simulink model "current"  (R2016b)
settings: Solver=VariableStepAuto  StartTime=0.0  StopTime=0.15  FixedStep=1e-5  MaxStep=Ts  RelTol=1e-4
model workspace (MAT data in the model file):
  TL = 0
  Ti = 0.001
  fpwm = 5000
  ts = 2e-06
undefined symbols (not defined in the file): Kii, Kpi, pmsm, Ts
libraries: nesl_utility x11, fl_lib x9, pe_lib x4, simulink x3, elec_lib x1, pePwmGeneratorTwoLevel x1
settings Model: Creator=25097  LastModifiedBy=25097
settings DebuggingCC: AlgebraicLoopMsg=error  ArtificialAlgebraicLoopMsg=error

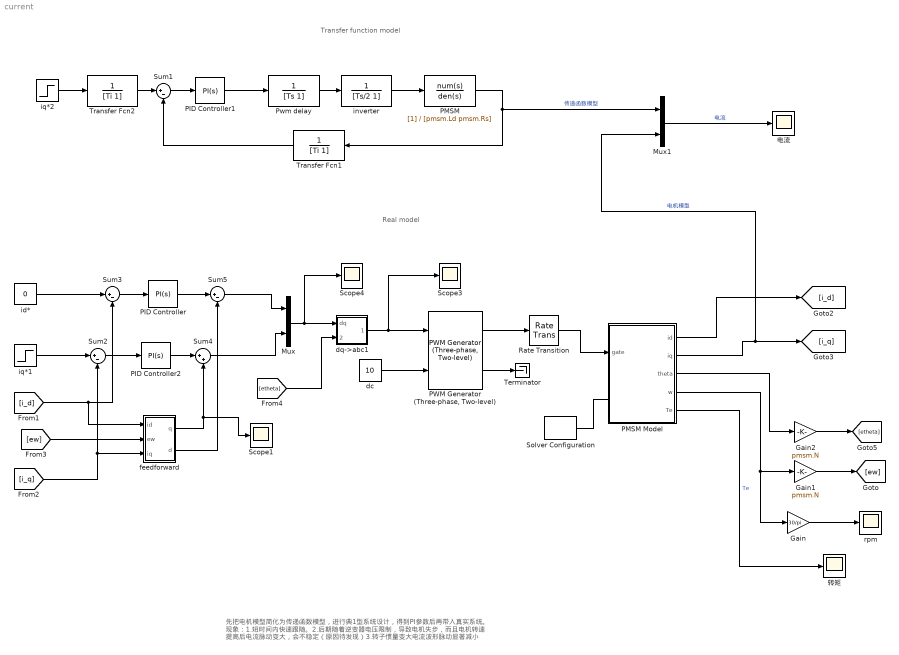
== system current ==
  note: 先把电机模型简化为传递函数模型，进行典1型系统设计，得到PI参数后再带入真实系统。
      | 现象：1.短时间内快速跟随。2.后期随着逆变器电压限制，导致电机失步，而且电机转速
      | 提高后电流脉动变大，会不稳定（原因待发现）3.转子惯量变大电流波形脉动显著减小
  note: Transfer function model
  note: Real model
  Gain : Gain  Gain=30/pi
  Gain1 : Gain  Gain=pmsm.N
  Gain2 : Gain  Gain=pmsm.N
  Mux : Mux  Inputs=2
  Mux1 : Mux  Inputs=2
  PID Controller : simulink/Continuous/PID Controller  Controller=PI  TimeDomain=Continuous-time  SampleTime=-1  IntegratorMethod=Forward Euler  FilterMethod=Forward Euler  Form=Parallel  UseFilter=on  ControllerParametersSource=internal  P=Kpi  I=Kii  D=0  N=100  InitialConditionSource=internal  InitialConditionForIntegrator=0  InitialConditionForFilter=0  ExternalReset=none  LimitOutput=off  UpperSaturationLimit=inf  LowerSaturationLimit=-inf  LinearizeAsGain=on  AntiWindupMode=none  Kb=1  TrackingMode=off  Kt=1  PParamMin=[]  PParamMax=[]  IParamMin=[]  IParamMax=[]  DParamMin=[]  DParamMax=[]  NParamMin=[]  NParamMax=[]  KbParamMin=[]  KbParamMax=[]  KtParamMin=[]  KtParamMax=[]  POutMin=[]  POutMax=[]  IOutMin=[]  IOutMax=[]  DOutMin=[]  DOutMax=[]  NOutMin=[]  NOutMax=[]  KbOutMin=[]  KbOutMax=[]  KtOutMin=[]  KtOutMax=[]  IntegratorOutMin=[]  IntegratorOutMax=[]  FilterOutMin=[]  FilterOutMax=[]  SumOutMin=[]  SumOutMax=[]  SumI1OutMin=[]  SumI1OutMax=[]  SumI2OutMin=[]  SumI2OutMax=[]  SumI3OutMin=[]  SumI3OutMax=[]  SumDOutMin=[]  SumDOutMax=[]  SaturationOutMin=[]  SaturationOutMax=[]  IntegratorContinuousStateAttributes=''  IntegratorStateMustResolveToSignalObject=off  IntegratorRTWStateStorageClass=Auto  FilterContinuousStateAttributes=''  FilterStateMustResolveToSignalObject=off  FilterRTWStateStorageClass=Auto  DifferentiatorICPrevScaledInput=0  DifferentiatorOutMin=[]  DifferentiatorOutMax=[]
  PID Controller1 : simulink/Continuous/PID Controller  Controller=PI  TimeDomain=Continuous-time  SampleTime=-1  IntegratorMethod=Forward Euler  FilterMethod=Forward Euler  Form=Parallel  UseFilter=on  ControllerParametersSource=internal  P=Kpi  I=Kii  D=0  N=100  InitialConditionSource=internal  InitialConditionForIntegrator=0  InitialConditionForFilter=0  ExternalReset=none  LimitOutput=off  UpperSaturationLimit=5  LowerSaturationLimit=-5  LinearizeAsGain=on  AntiWindupMode=none  Kb=1  TrackingMode=off  Kt=1  PParamMin=[]  PParamMax=[]  IParamMin=[]  IParamMax=[]  DParamMin=[]  DParamMax=[]  NParamMin=[]  NParamMax=[]  KbParamMin=[]  KbParamMax=[]  KtParamMin=[]  KtParamMax=[]  POutMin=[]  POutMax=[]  IOutMin=[]  IOutMax=[]  DOutMin=[]  DOutMax=[]  NOutMin=[]  NOutMax=[]  KbOutMin=[]  KbOutMax=[]  KtOutMin=[]  KtOutMax=[]  IntegratorOutMin=[]  IntegratorOutMax=[]  FilterOutMin=[]  FilterOutMax=[]  SumOutMin=[]  SumOutMax=[]  SumI1OutMin=[]  SumI1OutMax=[]  SumI2OutMin=[]  SumI2OutMax=[]  SumI3OutMin=[]  SumI3OutMax=[]  SumDOutMin=[]  SumDOutMax=[]  SaturationOutMin=[]  SaturationOutMax=[]  IntegratorContinuousStateAttributes=''  IntegratorStateMustResolveToSignalObject=off  IntegratorRTWStateStorageClass=Auto  FilterContinuousStateAttributes=''  FilterStateMustResolveToSignalObject=off  FilterRTWStateStorageClass=Auto  DifferentiatorICPrevScaledInput=0  DifferentiatorOutMin=[]  DifferentiatorOutMax=[]
  PID Controller2 : simulink/Continuous/PID Controller  Controller=PI  TimeDomain=Continuous-time  SampleTime=-1  IntegratorMethod=Forward Euler  FilterMethod=Forward Euler  Form=Parallel  UseFilter=on  ControllerParametersSource=internal  P=Kpi  I=Kii  D=0  N=100  InitialConditionSource=internal  InitialConditionForIntegrator=0  InitialConditionForFilter=0  ExternalReset=none  LimitOutput=off  UpperSaturationLimit=inf  LowerSaturationLimit=-inf  LinearizeAsGain=on  AntiWindupMode=none  Kb=1  TrackingMode=off  Kt=1  PParamMin=[]  PParamMax=[]  IParamMin=[]  IParamMax=[]  DParamMin=[]  DParamMax=[]  NParamMin=[]  NParamMax=[]  KbParamMin=[]  KbParamMax=[]  KtParamMin=[]  KtParamMax=[]  POutMin=[]  POutMax=[]  IOutMin=[]  IOutMax=[]  DOutMin=[]  DOutMax=[]  NOutMin=[]  NOutMax=[]  KbOutMin=[]  KbOutMax=[]  KtOutMin=[]  KtOutMax=[]  IntegratorOutMin=[]  IntegratorOutMax=[]  FilterOutMin=[]  FilterOutMax=[]  SumOutMin=[]  SumOutMax=[]  SumI1OutMin=[]  SumI1OutMax=[]  SumI2OutMin=[]  SumI2OutMax=[]  SumI3OutMin=[]  SumI3OutMax=[]  SumDOutMin=[]  SumDOutMax=[]  SaturationOutMin=[]  SaturationOutMax=[]  IntegratorContinuousStateAttributes=''  IntegratorStateMustResolveToSignalObject=off  IntegratorRTWStateStorageClass=Auto  FilterContinuousStateAttributes=''  FilterStateMustResolveToSignalObject=off  FilterRTWStateStorageClass=Auto  DifferentiatorICPrevScaledInput=0  DifferentiatorOutMin=[]  DifferentiatorOutMax=[]
  "PMSM " : TransferFcn  Denominator=[pmsm.Ld pmsm.Rs]
  PMSM Model : Subsystem
      settings: MinAlgLoopOccurrences=on
  "PWM Generator (Three-phase, Two-level)" : pePwmGeneratorTwoLevel/PWM Generator (Three-phase, Two-level)  OverrideUsingVariant=NaturalMode  PWMMode=Continuous PWM (CPWM)  CPWMMode=SPWM: sinusoidal PWM  DPWMMode=60 DPWM: 60 degree discontinuous PWM  fsw=fpwm  Ts=ts
      settings: SamplingMode=Natural
  "Pwm delay " : TransferFcn  Denominator=[Ts 1]
  Rate Transition : RateTransition
  Scope1 : Scope
  Scope3 : Scope
  Scope4 : Scope
  Solver Configuration : nesl_utility/Solver Configuration  PhysicalDomain=network_engine_domain  SubClassName=solver  LeftPortType=input  RightPortType=generic  Accelerate=off  Tones=[]  Harmonics=[]  SimulateNoise=off  Profile=off  UseLocalSampling=off  EnableSwitchedLinearOptims=on  FrequencyDomain=off  UseCCode=off  RelTol=0.001  AbsTol=1e-06  MinStep=1e-09  ToWorkspace=off  RevertToSquareIcSolve=off  NumHomotopyIterations=100  PhasorMode=off  PhasorModeNumHarmonics=1  OverrideAbsTol=off  DoDC=off  ResidualTolerance=1e-07  UseLocalSolver=off  LocalSolverChoice=NE_BACKWARD_EULER_ADVANCER  LocalSolverSampleTime=1e-6  DoFixedCost=off  MaxNonlinIter=3  MaxModeIter=2  LinearAlgebra=Sparse  DelaysMemoryBudget=1024  AutomaticFiltering=on  FilteringTimeConstant=0.001
  Sum{1..3,5} (4 alike) : Sum  Inputs=|+-
  Sum4 : Sum  Inputs=|++
  Terminator : Terminator
  Transfer Fcn1 : TransferFcn  Denominator=[Ti 1]
  Transfer Fcn2 : TransferFcn  Denominator=[Ti 1]
  dc : Constant  Value=10
  dq->abc1 : Subsystem
  "feedforward " : Subsystem
  id* : Constant  Value=0
  inverter : TransferFcn  Denominator=[Ts/2 1]
  iq*1 : Step  Time=0.05  After=3  SampleTime=0
  iq*2 : Step  Time=0.05  After=3  SampleTime=0
  rpm : Scope
  电流 : Scope
  转矩 : Scope
  wires:
  iq*2/1 -> Transfer Fcn2/1
  Transfer Fcn2/1 -> Sum1/1
  Sum1/1 -> PID Controller1/1
  PID Controller1/1 -> "Pwm delay "/1
  "Pwm delay "/1 -> inverter/1
  inverter/1 -> "PMSM "/1
  "PMSM "/1 -> Mux1/1, Transfer Fcn1/1  "传递函数模型"
  Transfer Fcn1/1 -> Sum1/2
  iq*1/1 -> Sum2/1
  Sum2/1 -> PID Controller2/1
  PID Controller2/1 -> Sum4/1
  id*/1 -> Sum3/1
  Sum3/1 -> PID Controller/1
  PID Controller/1 -> Sum5/1
  "feedforward "/1(q) -> Sum4/2, Scope1/1
  "feedforward "/2(d) -> Sum5/2
  [ew] -> "feedforward "/2(ew)
  Sum4/1 -> Mux/2
  Sum5/1 -> Mux/1
  Mux/1 -> Scope4/1, dq->abc1/1(dq)
  [etheta] -> dq->abc1/2("theta ")
  dc/1 -> "PWM Generator (Three-phase, Two-level)"/2
  "PWM Generator (Three-phase, Two-level)"/2 -> Terminator/1
  PMSM Model/3(theta) -> Gain2/1
  Mux1/1 -> 电流/1  "电流"
  Gain/1 -> rpm/1
  PMSM Model/5("Te ") -> 转矩/1  "Te"
  PMSM Model/4(w) -> Gain1/1, Gain/1
  Gain2/1 -> [etheta]
  Gain1/1 -> [ew]
  PMSM Model/1(id) -> [i_d]
  PMSM Model/2(iq) -> Mux1/2, [i_q]  "电机模型"
  [i_d] -> "feedforward "/1("id "), Sum3/2
  [i_q] -> "feedforward "/3(iq), Sum2/2
  dq->abc1/1(abc) -> Scope3/1, "PWM Generator (Three-phase, Two-level)"/1
  "PWM Generator (Three-phase, Two-level)"/1 -> Rate Transition/1
  Rate Transition/1 -> PMSM Model/1("gate ")
  connections:
  Solver Configuration/RConn1 -- PMSM Model/LConn1

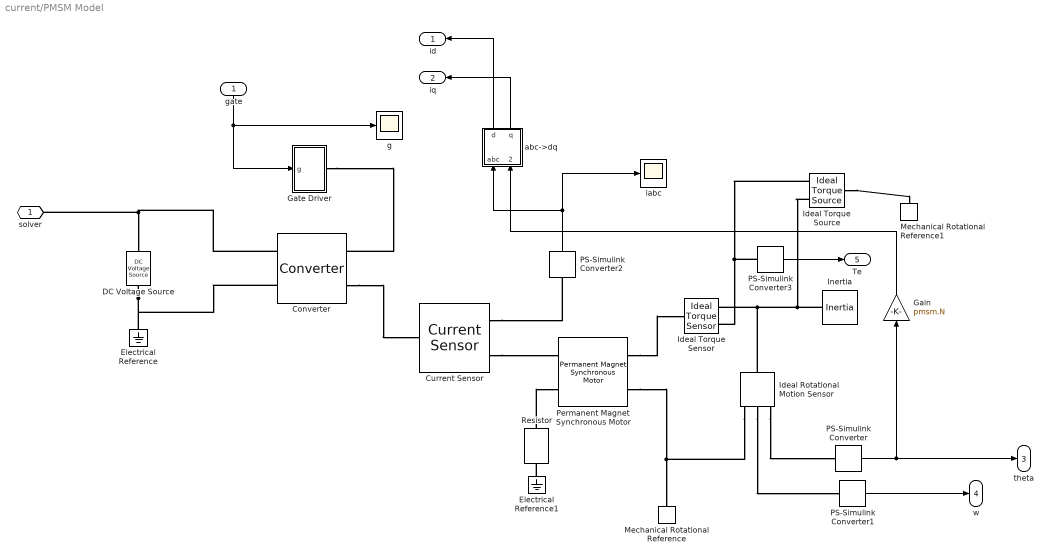
== system current/PMSM Model ==
  "gate " : Inport
  Converter : pe_lib/Semiconductors/Converter  device_type=2  Vf=0.8 V  Ron=0.001 Ohm  Rds=0.001 Ohm  Goff=1e-8 1/Ohm  Vth=0.5 V  Vgt=1 V  Vgt_off=-1 V  Ih=1 A  diode_param=1  diode_Vf=0.8 V  diode_Ron=0.001 Ohm  diode_Goff=1e-5 1/Ohm  diode_C=50 nF  diode_iRM=-235 A  diode_iF=300 A  diode_idot=-50 A/us  diode_trr_param=1  diode_trr_factor=3  diode_trr=15 us  diode_Qrr=1.5e+3 s*uA  snubber_type=0  Rs=0.1 Ohm  Cs=1e-7 F
  Current Sensor : pe_lib/Sensors/Current Sensor
  DC Voltage Source : elec_lib/Additional Components/SPICE-Compatible Components/Sources/DC Voltage Source  DC=10 V
  Electrical Reference : fl_lib/Electrical/Electrical Elements/Electrical Reference
  Electrical Reference1 : fl_lib/Electrical/Electrical Elements/Electrical Reference
  Gain : Gain  Gain=pmsm.N
  Gate Driver : Subsystem
  Ideal Rotational Motion Sensor : fl_lib/Mechanical/Mechanical Sensors/Ideal Rotational Motion Sensor  offset=0 rad
  Ideal Torque Sensor : fl_lib/Mechanical/Mechanical Sensors/Ideal Torque Sensor
  Ideal Torque Source : fl_lib/Mechanical/Mechanical Sources/Ideal Torque Source
  Inertia : fl_lib/Mechanical/Rotational Elements/Inertia  inertia=pmsm.J kg*m^2  w_specify=off  w_priority=High  w=0 rad/s  t_specify=off  t_priority=None  t=0 N*m
  Mechanical Rotational Reference : fl_lib/Mechanical/Rotational Elements/Mechanical Rotational Reference
  Mechanical Rotational Reference1 : fl_lib/Mechanical/Rotational Elements/Mechanical Rotational Reference
  PS-Simulink Converter{,1..3} (4 alike) : nesl_utility/PS-Simulink Converter  PhysicalDomain=network_engine_domain  SubClassName=ps_output  LeftPortType=input  RightPortType=output  PseudoPeriodic=off  Frequencies=[]  Unit=1  AffineConversion=off
  Permanent Magnet Synchronous Motor : pe_lib/Machines/Permanent Magnet Rotor/Permanent Magnet Synchronous Motor  nPolePairs=pmsm.N  pm_flux_linkage=pmsm.PM Wb  stator_param=1  Ld=pmsm.Ld H  Lq=pmsm.Ld H  L0=pmsm.Ld H  Ls=0.0002 H  Lm=0.00002 H  Ms=0.00002 H  Rs=pmsm.Rs Ohm  initial_currents=[0.0, 0.0, 0.0] A  axes_param=2  angular_position0=0 rad  rotor_offset=-pi / 2 rad  shift_3ph=[nan, nan, nan] rad  sqrt2OverSqrt3=nan  oneOverSqrt2=nan  twoPiOver3=nan  Lmin=1e-9 H
  Resistor : fl_lib/Electrical/Electrical Elements/Resistor  R=1e9 Ohm  i_specify=off  i_priority=None  i=0 A  v_specify=off  v_priority=None  v=0 V
  abc->dq : Subsystem
  g : Scope
  iabc : Scope
  "solver " : PMIOPort  Port=1  Side=Left
  id : Outport
  iq : Outport  Port=2
  theta : Outport  Port=3
  w : Outport  Port=4
  "Te " : Outport  Port=5
  wires:
  PS-Simulink Converter/1 -> Gain/1, theta/1
  PS-Simulink Converter2/1 -> abc->dq/1(abc), iabc/1
  PS-Simulink Converter1/1 -> w/1
  abc->dq/1(d) -> id/1
  abc->dq/2(q) -> iq/1
  PS-Simulink Converter3/1 -> "Te "/1
  Gain/1 -> abc->dq/2(theta)
  "gate "/1 -> g/1, Gate Driver/1(g)
  connections:
  DC Voltage Source/RConn1 -- Electrical Reference/LConn1 -- Converter/RConn2
  Converter/RConn1 -- DC Voltage Source/LConn1 -- "solver "/RConn1
  Current Sensor/RConn1 -- PS-Simulink Converter2/LConn1
  Converter/LConn2 -- Current Sensor/LConn1
  Resistor/LConn1 -- Permanent Magnet Synchronous Motor/LConn2
  Current Sensor/RConn2 -- Permanent Magnet Synchronous Motor/LConn1
  Electrical Reference1/LConn1 -- Resistor/RConn1
  Gate Driver/RConn1 -- Converter/LConn1
  Permanent Magnet Synchronous Motor/RConn2 -- Mechanical Rotational Reference/LConn1 -- Ideal Rotational Motion Sensor/RConn1
  Permanent Magnet Synchronous Motor/RConn1 -- Ideal Torque Sensor/LConn1
  Inertia/LConn1 -- Ideal Torque Source/RConn2 -- Ideal Rotational Motion Sensor/LConn1 -- Ideal Torque Sensor/RConn1
  Ideal Rotational Motion Sensor/RConn3 -- PS-Simulink Converter/LConn1
  Ideal Rotational Motion Sensor/RConn2 -- PS-Simulink Converter1/LConn1
  PS-Simulink Converter3/LConn1 -- Ideal Torque Source/RConn1 -- Ideal Torque Sensor/RConn2
  Ideal Torque Source/LConn1 -- Mechanical Rotational Reference1/LConn1

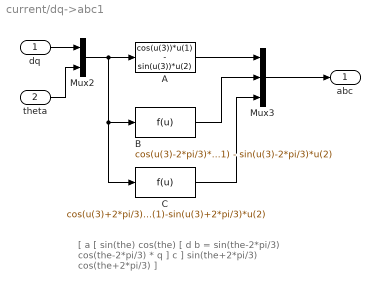
== system current/dq->abc1 ==
  note: [ a        [  sin(the)               cos(the)                 [ d
      |
      |   b    =     sin(the-2*pi/3)    cos(the-2*pi/3)    *    q ]
      |
      |   c ]         sin(the+2*pi/3)   cos(the+2*pi/3) ]
  dq : Inport
  "theta " : Inport  Port=2
  A : Fcn  Expr=cos(u(3))*u(1) - sin(u(3))*u(2)
  B : Fcn  Expr=cos(u(3)-2*pi/3)*u(1) - sin(u(3)-2*pi/3)*u(2)
  C : Fcn  Expr=cos(u(3)+2*pi/3)*u(1)-sin(u(3)+2*pi/3)*u(2)
  Mux2 : Mux  Inputs=2
  Mux3 : Mux  Inputs=3
  abc : Outport
  wires:
  Mux3/1 -> abc/1
  C/1 -> Mux3/3
  A/1 -> Mux3/1
  dq/1 -> Mux2/1
  "theta "/1 -> Mux2/2
  Mux2/1 -> C/1, B/1, A/1
  B/1 -> Mux3/2

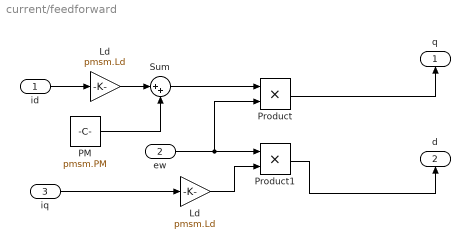
== system current/feedforward  ==
  "id " : Inport
  ew : Inport  Port=2
  iq : Inport  Port=3
  Ld : Gain  Gain=pmsm.Ld
  "Ld " : Gain  Gain=pmsm.Ld
  PM : Constant  Value=pmsm.PM
  Product : Product
  Product1 : Product
  Sum : Sum  Inputs=|++
  q : Outport
  d : Outport  Port=2
  wires:
  "id "/1 -> Ld/1
  PM/1 -> Sum/2
  Ld/1 -> Sum/1
  "Ld "/1 -> Product1/2
  Product/1 -> q/1
  Sum/1 -> Product/1
  Product1/1 -> d/1
  iq/1 -> "Ld "/1
  ew/1 -> Product1/1, Product/2

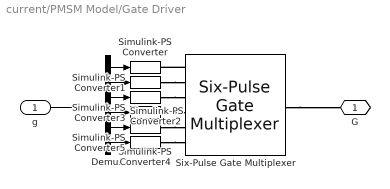
== system current/PMSM Model/Gate Driver ==
  g : Inport
  Demux : Demux  Outputs=6
  Simulink-PS Converter{,1..5} (6 alike) : nesl_utility/Simulink-PS Converter  PhysicalDomain=network_engine_domain  SubClassName=ps_input  LeftPortType=input  RightPortType=output  PseudoPeriodic=off  Frequencies=[]  NoiseDistribution=none  NoiseParameters=[]  Unit=1  AffineConversion=off  InputFiltering=off  SimscapeFilterOrder=1  InputFilterTimeConstant=0.001  UdotUserProvided=1
  Six-Pulse Gate Multiplexer : pe_lib/Semiconductors/Six-Pulse Gate Multiplexer  R=0 Ohm
  G : PMIOPort  Port=1  Side=Right
  wires:
  g/1 -> Demux/1
  Demux/1 -> Simulink-PS Converter/1
  Demux/2 -> Simulink-PS Converter1/1
  Demux/3 -> Simulink-PS Converter2/1
  Demux/4 -> Simulink-PS Converter3/1
  Demux/5 -> Simulink-PS Converter4/1
  Demux/6 -> Simulink-PS Converter5/1
  connections:
  Six-Pulse Gate Multiplexer/LConn1 -- Simulink-PS Converter/RConn1
  Simulink-PS Converter1/RConn1 -- Six-Pulse Gate Multiplexer/LConn2
  Simulink-PS Converter2/RConn1 -- Six-Pulse Gate Multiplexer/LConn3
  Simulink-PS Converter3/RConn1 -- Six-Pulse Gate Multiplexer/LConn4
  Simulink-PS Converter4/RConn1 -- Six-Pulse Gate Multiplexer/LConn5
  Simulink-PS Converter5/RConn1 -- Six-Pulse Gate Multiplexer/LConn6
  Six-Pulse Gate Multiplexer/RConn1 -- G/RConn1

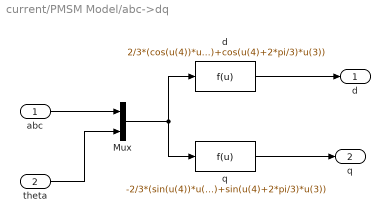
== system current/PMSM Model/abc->dq ==
  abc : Inport
  theta : Inport  Port=2
  Mux : Mux  Inputs=2
  "d " : Fcn  Expr=2/3*(cos(u(4))*u(1)+cos(u(4)-2*pi/3)*u(2)+cos(u(4)+2*pi/3)*u(3))
  "q " : Fcn  Expr=-2/3*(sin(u(4))*u(1)+sin(u(4)-2*pi/3)*u(2)+sin(u(4)+2*pi/3)*u(3))
  d : Outport
  q : Outport  Port=2
  wires:
  "d "/1 -> d/1
  "q "/1 -> q/1
  abc/1 -> Mux/1
  Mux/1 -> "q "/1, "d "/1
  theta/1 -> Mux/2
